simulink model "DAB_Tri_Trap"  (R2022b)
settings: Solver=ode23t  StartTime=0.0  StopTime=1/fsw*10000  MaxStep=1/100000  RelTol=1e-7  AbsTol=1e-7
StartFcn:
  | tic
StopFcn:
  | toc
undefined symbols (not defined in the file): DiscIntNeverNeededParam, fsw, L, n, ntemp, period, R_Load, tau, ts_pwm, Vdc1, Vth
libraries: nesl_utility x15, fl_lib x12, ee_lib x8, simulink x5, slpidlib x1
(part 1 of 2)
settings Model: Creator=jvansick  LastModifiedBy=jvansick
settings SolverCC: AutoScaleAbsTol=off  ExtrapolationOrder=1  ODENIntegrationMethod=ode14x
settings DebuggingCC: UnconnectedInputMsg=warning  UnconnectedOutputMsg=warning  UnconnectedLineMsg=warning
settings ModelReferenceCC: EnableRefExpFcnMdlSchedulingChecks=on
settings RTWCC: DLArmComputeVersion=19.05

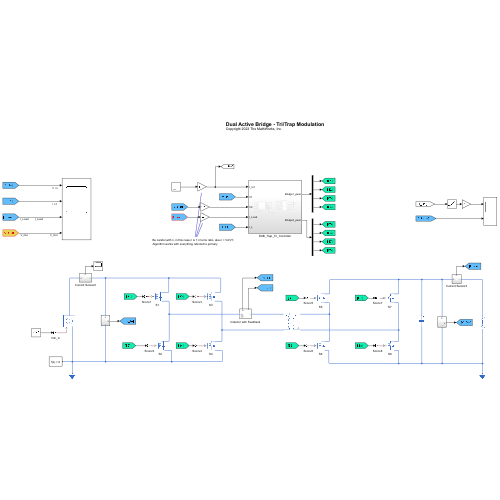
[thumbnail: Simulink's stored preview of the top-level diagram]
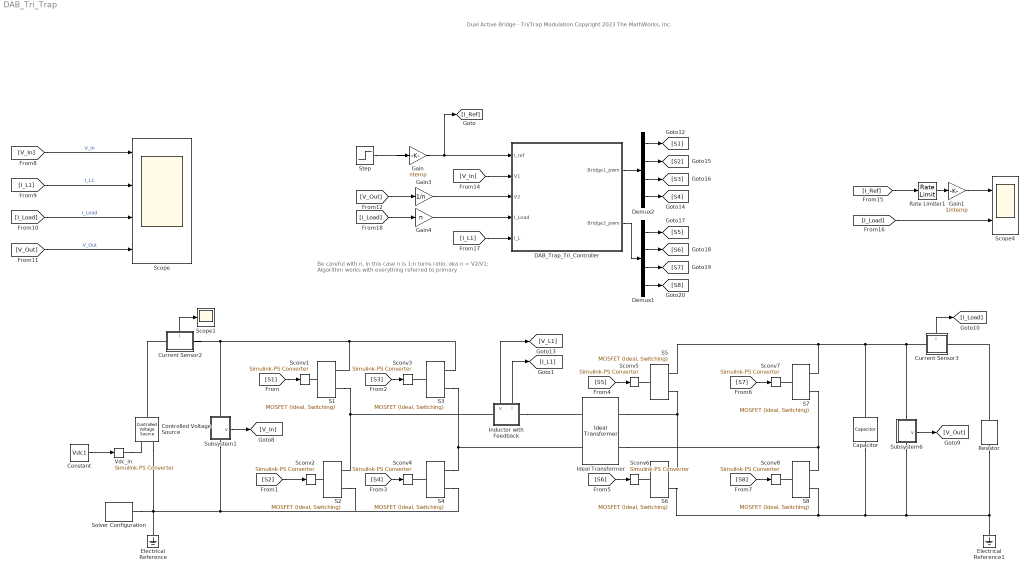
== system DAB_Tri_Trap ==
  note: Be careful with n, in this case n is 1:n turns ratio, aka n = V2/V1; Algorithm works with everything referred to primary
  note: Dual Active Bridge - Tri/Trap Modulation
      | Copyright 2023 The MathWorks, Inc.
  Capacitor : fl_lib/Electrical/Electrical Elements/Capacitor  c=Cout F  r=0 Ohm  g=0 1/Ohm  i_specify=off  i_priority=None  i=0 A  i_nominal_specify=off  i_nominal_unit=A  i_nominal_value=1  v_specify=off  v_priority=None  v=Vdc2 V  v_nominal_specify=off  v_nominal_unit=V  v_nominal_value=1  vc_specify=on  vc_priority=High  vc=Vdc2 V  vc_nominal_specify=off  vc_nominal_unit=V  vc_nominal_value=1
  Constant : Constant  Value=Vdc1
  Controlled Voltage Source : fl_lib/Electrical/Electrical Sources/Controlled Voltage Source
  Current Sensor2 : Subsystem
      settings: PortSchema="{\"entries\":[{\"content\":{\"sides\":[{\"content\":{\"connectorIds\":[\"LConn1\"]},\"type\":\"ConnectorPlacement.EquallySpacedRectSide\",\"uuid\":\"e9388151-e471-4783-81c5-5134e1313d7c\"},{\"content\":{\"connectorIds\":[\"RConn1\"],\"side\":\"RIGHT\"},\"type\":\"ConnectorPlacement.EquallySpacedRectSide\",\"uuid\":\"bcb23f28-0826-4736-ab91-150a314eb643\"},{\"content\":{\"connectorIds\":[\"Out1\"],\"side\":\"TOP\"},\"type\":\"ConnectorPlacement.EquallySpacedRectSide\",\"uuid\":\"e1937689-3337-4922-a316-f56c73fb0974\"}]},\"type\":\"ConnectorPlacement.EquallySpacedConnector\",\"uuid\":\"dc34a384-5aa5-46fc-88a5-47651899efae\"}],\"packageUris\":[\"http://schema.mathworks.com/mf0/Connector/R2020b\"],\"version\":\"1.0\"}"
  Current Sensor3 : Subsystem
      settings: PortSchema="{\"entries\":[{\"content\":{\"sides\":[{\"content\":{\"connectorIds\":[\"LConn1\"]},\"type\":\"ConnectorPlacement.EquallySpacedRectSide\",\"uuid\":\"e9388151-e471-4783-81c5-5134e1313d7c\"},{\"content\":{\"connectorIds\":[\"RConn1\"],\"side\":\"RIGHT\"},\"type\":\"ConnectorPlacement.EquallySpacedRectSide\",\"uuid\":\"bcb23f28-0826-4736-ab91-150a314eb643\"},{\"content\":{\"connectorIds\":[\"Out1\"],\"side\":\"TOP\"},\"type\":\"ConnectorPlacement.EquallySpacedRectSide\",\"uuid\":\"e1937689-3337-4922-a316-f56c73fb0974\"}]},\"type\":\"ConnectorPlacement.EquallySpacedConnector\",\"uuid\":\"dc34a384-5aa5-46fc-88a5-47651899efae\"}],\"packageUris\":[\"http://schema.mathworks.com/mf0/Connector/R2020b\"],\"version\":\"1.0\"}"
  DAB_Trap_Tri_Controller : Subsystem
  Demux1 : Demux
  Demux2 : Demux
  Electrical Reference : fl_lib/Electrical/Electrical Elements/Electrical Reference
  Electrical Reference1 : fl_lib/Electrical/Electrical Elements/Electrical Reference
  Gain : Gain  Gain=ntemp
  Gain1 : Gain  Gain=1/ntemp
  Gain3 : Gain  Gain=1/n
  Gain4 : Gain  Gain=n
  Ideal Transformer : fl_lib/Electrical/Electrical Elements/Ideal Transformer  n=1/n  i1_specify=off  i1_priority=None  i1=0 A  i1_nominal_specify=off  i1_nominal_unit=A  i1_nominal_value=1  v1_specify=off  v1_priority=None  v1=0 V  v1_nominal_specify=off  v1_nominal_unit=V  v1_nominal_value=1  i2_specify=off  i2_priority=None  i2=0 A  i2_nominal_specify=off  i2_nominal_unit=A  i2_nominal_value=1  v2_specify=off  v2_priority=None  v2=0 V  v2_nominal_specify=off  v2_nominal_unit=V  v2_nominal_value=1
  Inductor with Feedback : Subsystem  mask{L=L}
      mask prompts: L "Inductance"
      settings: PortSchema="{\"entries\":[{\"content\":{\"sides\":[{\"content\":{\"connectorIds\":[\"LConn1\"]},\"type\":\"ConnectorPlacement.EquallySpacedRectSide\",\"uuid\":\"d17b03de-5a5d-44ef-b1c9-12c97ac90336\"},{\"content\":{\"connectorIds\":[\"RConn1\"],\"side\":\"RIGHT\"},\"type\":\"ConnectorPlacement.EquallySpacedRectSide\",\"uuid\":\"dcf9dd19-1bc3-435d-be19-5082ce08996a\"},{\"content\":{\"connectorIds\":[\"Out1\",\"Out2\"],\"side\":\"TOP\"},\"type\":\"ConnectorPlacement.EquallySpacedRectSide\",\"uuid\":\"d1169a59-8047-479a-baab-e2604a43bf69\"}]},\"type\":\"ConnectorPlacement.EquallySpacedConnector\",\"uuid\":\"f70215f2-dcac-493e-85d0-6d9635986165\"}],\"packageUris\":[\"http://schema.mathworks.com/mf0/Connector/R2020b\"],\"version\":\"1.0\"}"
  Rate Limiter1 : RateLimiter  RisingSlewLimit=fsw/500  FallingSlewLimit=-fsw/500  SampleTimeMode=inherited  InitialCondition=15*ntemp
  Resistor : fl_lib/Electrical/Electrical Elements/Resistor  R=R_Load Ohm  i_specify=off  i_priority=None  i=0 A  i_nominal_specify=off  i_nominal_unit=A  i_nominal_value=1  v_specify=off  v_priority=None  v=0 V  v_nominal_specify=off  v_nominal_unit=V  v_nominal_value=1
  S{1..8} (8 alike) : ee_lib/Semiconductors & Converters/MOSFET (Ideal, Switching)  port_option=ee.enum.controlport.ps  Rds=R_ds Ohm  Goff=1e-5 1/Ohm  Vth=Vth V  diode_param=2  diode_Vf=V_fw_d V  diode_Ron=R_don Ohm  diode_Goff=1e-5 1/Ohm  diode_C=50e-9 F  diode_iRM=-235 A  diode_iF=300 A  diode_idot=-50 A/us  diode_trr_param=1  diode_trr_factor=3  diode_trr=15 us  diode_Qrr=1500 s*uA  ids_specify=off  ids_priority=None  ids=0 A  ids_nominal_specify=off  ids_nominal_unit=A  ids_nominal_value=1  vds_specify=off  vds_priority=None  vds=0 V  vds_nominal_specify=off  vds_nominal_unit=V  vds_nominal_value=1  vgs_specify=off  vgs_priority=None  vgs=0 V  vgs_nominal_specify=off  vgs_nominal_unit=V  vgs_nominal_value=1  thermal_loss_option=ee.enum.converters.thermalLossOption.constantvalues  Von_data=[0, 1.8, 3.2, 6, 10, 16; 0, 2, 5.5, 9.5, 15, 25] V  Tj=[298.15, 448.15] K  Iout_data=[0, 20, 40, 60, 80, 100] A  Eon_data=[0, 55.04, 124.57, 235.53, 362.12; 0, 71.25, 161.25, 304.88, 468.75] * 1e-6 J  Eoff_data=[0, 18, 30, 56.1, 76.5; 0, 22.5, 37.5, 70.13, 95.63] * 1e-6 J  Tj_loss=[298.15, 448.15] K  Iout_data_loss=[0, 10, 20, 30, 40] A  Eon_scalar=22.86e-3 J  Eoff_scalar=17.14e-3 J  Voff=300 V  Iout_scalar=600 A  diodeModelType=ee.enum.converters.diodeModelType.pwl  diodeTableType=ee.enum.diode.tableType.IfMat  diode_IfMat=[.07, .12, .19, 1.75, 4.24, 7.32, 11.2; .16, .3, .72, 2.14, 4.02, 6.35, 9.12] A  diode_VfMat=[.9, 1.15, 1.25, 1.5, 1.75, 2.17, 2.6, 2.85; .58, .68, .75, 1.1, 1.38, 1.77, 2.27, 2.7] V  diode_TjVec=[25, 125] degC  diode_VfVec=[.5, .7, .9, 1.3, 1.7, 2.1, 2.5] V  diode_IfVec=[.1, .2, .5, 1, 2, 4, 7, 10] A  diode_Vr=-600 V  diode_Ls=150 nH  diode_Erec=0.03 J  thermal_network_parameterization=ee.enum.thermalNetworkTopology.external  Rth=[.03, .2] K/W  Rth_Cauer=[.03, .1, .2] K/W  Rth_Foster=[.03, .2] K/W  thermal_mass_parameterization=ee.enum.thermalNetwork.timeconstant  thermal_mass=[3, 25] J/K  thermal_mass_Cauer=[3, 10, 25] J/K  thermal_mass_Foster=[33, 50] J/K  thermal_time_constant=[.1, 5] s  thermal_time_constant_Cauer=[.1, 1, 5] s  thermal_time_constant_Foster=[1, 10] s  thermal_mass_initial_temperatures=[25, 25] degC  thermal_mass_initial_temperatures_Cauer=[25, 25, 25] degC  junction_thermal_mass=0.1 J/K  Tvec_initial_Foster=[25, 25, 25, 25] degC  no_thermal_network=0  junction_temperature_specify=off  junction_temperature_priority=None  junction_temperature=25 degC  junction_temperature_nominal_specify=off  junction_temperature_nominal_unit=degC  junction_temperature_nominal_value=1  Qj_specify=off  Qj_priority=None  Qj=0 W  Qj_nominal_specify=off  Qj_nominal_unit=W  Qj_nominal_value=1
  Sconv{1..8} (8 alike) : nesl_utility/Simulink-PS Converter  PhysicalDomain=network_engine_domain  SubClassName=ps_input  LeftPortType=input  RightPortType=output  PseudoPeriodic=off  Frequencies=[]  NoiseDistribution=none  NoiseParameters=[]  Unit=1  AffineConversion=off  FilteringAndDerivatives=provide  SimscapeFilterOrder=1  InputFilterTimeConstant=0.001  UdotUserProvided=0
  Scope : Scope  NumInputPorts=4
  Scope1 : Scope
  Scope4 : Scope  NumInputPorts=2
  Solver Configuration : nesl_utility/Solver Configuration  PhysicalDomain=network_engine_domain  SubClassName=solver  LeftPortType=input  RightPortType=generic  Tones=[]  Harmonics=[]  SimulateNoise=off  Profile=off  UseLocalSampling=off  EnableSwitchedLinearOptims=on  FrequencyDomain=off  UseCCode=off  RelTol=0.001  AbsTol=1e-06  MinStep=1e-09  ToWorkspace=off  RevertToSquareIcSolve=off  NumHomotopyIterations=100  PhasorMode=off  PhasorModeNumHarmonics=1  ConsistencySolver=NEWTON_FTOL  IndexReductionMethod=DerivativeReplacement  DoDC=off  ResidualTolerance=1e-09  ConsistencyTolSource=GLOBAL  ConsistencyAbsTol=0.001  ConsistencyRelTol=0.001  ConsistencyTolFactor=0.001  UseLocalSolver=off  LocalSolverChoice=NE_BACKWARD_EULER_ADVANCER  ResolveIndetEquations=on  FunctionEvalNumThread=1  LocalSolverSampleTime=0.001  DoFixedCost=off  MaxNonlinIter=3  MaxModeIter=2  ComputeImpulses=off  ImpulseIterations=2  LinearAlgebra=auto  LinearAlgebraNumThread=0  EquationFormulation=NE_TIME_EF  DelaysMemoryBudget=1024  AutomaticFiltering=on  FilteringTimeConstant=0.001  PartitionStorageMethod=AS_NEEDED  PartitionMemoryBudget=1024  PartitionMethod=ROBUST
  Step : Step  Time=1/fsw*5000  Before=15.25  After=19.35  SampleTime=1/fsw
  Subsystem1 : Subsystem
      settings: PortSchema="{\"entries\":[{\"content\":{\"sides\":[{\"content\":{\"connectorIds\":[\"LConn1\"]},\"type\":\"ConnectorPlacement.EquallySpacedRectSide\",\"uuid\":\"e9388151-e471-4783-81c5-5134e1313d7c\"},{\"content\":{\"connectorIds\":[\"RConn1\"],\"side\":\"RIGHT\"},\"type\":\"ConnectorPlacement.EquallySpacedRectSide\",\"uuid\":\"bcb23f28-0826-4736-ab91-150a314eb643\"},{\"content\":{\"connectorIds\":[\"Out1\"],\"side\":\"TOP\"},\"type\":\"ConnectorPlacement.EquallySpacedRectSide\",\"uuid\":\"e1937689-3337-4922-a316-f56c73fb0974\"}]},\"type\":\"ConnectorPlacement.EquallySpacedConnector\",\"uuid\":\"dc34a384-5aa5-46fc-88a5-47651899efae\"}],\"packageUris\":[\"http://schema.mathworks.com/mf0/Connector/R2020b\"],\"version\":\"1.0\"}"
  Subsystem6 : Subsystem
      settings: PortSchema="{\"entries\":[{\"content\":{\"sides\":[{\"content\":{\"connectorIds\":[\"LConn1\"]},\"type\":\"ConnectorPlacement.EquallySpacedRectSide\",\"uuid\":\"e9388151-e471-4783-81c5-5134e1313d7c\"},{\"content\":{\"connectorIds\":[\"RConn1\"],\"side\":\"RIGHT\"},\"type\":\"ConnectorPlacement.EquallySpacedRectSide\",\"uuid\":\"bcb23f28-0826-4736-ab91-150a314eb643\"},{\"content\":{\"connectorIds\":[\"Out1\"],\"side\":\"TOP\"},\"type\":\"ConnectorPlacement.EquallySpacedRectSide\",\"uuid\":\"e1937689-3337-4922-a316-f56c73fb0974\"}]},\"type\":\"ConnectorPlacement.EquallySpacedConnector\",\"uuid\":\"dc34a384-5aa5-46fc-88a5-47651899efae\"}],\"packageUris\":[\"http://schema.mathworks.com/mf0/Connector/R2020b\"],\"version\":\"1.0\"}"
  Vdc_in : nesl_utility/Simulink-PS Converter  PhysicalDomain=network_engine_domain  SubClassName=ps_input  LeftPortType=input  RightPortType=output  PseudoPeriodic=off  Frequencies=[]  NoiseDistribution=none  NoiseParameters=[]  Unit=1  AffineConversion=off  FilteringAndDerivatives=provide  SimscapeFilterOrder=1  InputFilterTimeConstant=0.001  UdotUserProvided=0
  wires:
  [S1] -> Sconv1/1
  [S2] -> Sconv2/1
  [S3] -> Sconv3/1
  [S4] -> Sconv4/1
  [S6] -> Sconv6/1
  [S7] -> Sconv7/1
  [S8] -> Sconv8/1
  [S5] -> Sconv5/1
  Constant/1 -> Vdc_in/1
  Subsystem1/1(v) -> [V_In]
  [V_In] -> Scope/1  "V_in"
  [I_L1] -> Scope/2  "I_L1"
  [I_Load] -> Scope/3  "I_Load"
  Current Sensor2/1(i) -> Scope1/1
  [V_Out] -> Scope/4  "V_Out"
  Demux2/1 -> [S1]
  Demux2/4 -> [S4]
  Demux2/2 -> [S2]
  Demux2/3 -> [S3]
  Demux1/1 -> [S5]
  Demux1/2 -> [S6]
  Demux1/3 -> [S7]
  Demux1/4 -> [S8]
  DAB_Trap_Tri_Controller/2(Bridge2_pwm) -> Demux1/1
  DAB_Trap_Tri_Controller/1(Bridge1_pwm) -> Demux2/1
  Current Sensor3/1(i) -> [I_Load]
  Subsystem6/1(v) -> [V_Out]
  Step/1 -> Gain/1
  [V_Out] -> Gain3/1
  [V_In] -> DAB_Trap_Tri_Controller/2(V1)
  [I_L1] -> DAB_Trap_Tri_Controller/5(I_L)
  [I_Load] -> Gain4/1
  [I_Load] -> Scope4/2
  [I_Ref] -> Rate Limiter1/1
  Rate Limiter1/1 -> Gain1/1
  Gain/1 -> [I_Ref], DAB_Trap_Tri_Controller/1(I_ref)
  Gain3/1 -> DAB_Trap_Tri_Controller/3(V2)
  Gain4/1 -> DAB_Trap_Tri_Controller/4(I_Load)
  Inductor with Feedback/1(v) -> [V_L1]
  Inductor with Feedback/2(i) -> [I_L1]
  Gain1/1 -> Scope4/1
  connections:
  Subsystem1/LConn1 -- Current Sensor2/RConn1 -- S1/RConn1 -- S3/RConn1
  Controlled Voltage Source/RConn2 -- Electrical Reference/LConn1 -- S4/RConn2 -- S2/RConn2 -- Subsystem1/RConn1 -- Solver Configuration/RConn1
  Vdc_in/RConn1 -- Controlled Voltage Source/RConn1
  S2/LConn1 -- Sconv2/RConn1
  Sconv1/RConn1 -- S1/LConn1
  S3/LConn1 -- Sconv3/RConn1
  S4/LConn1 -- Sconv4/RConn1
  S6/LConn1 -- Sconv6/RConn1
  S8/LConn1 -- Sconv8/RConn1
  S7/LConn1 -- Sconv7/RConn1
  S5/LConn1 -- Sconv5/RConn1
  S3/RConn2 -- S4/RConn1 -- Ideal Transformer/LConn2
  S5/RConn2 -- Ideal Transformer/RConn1 -- S6/RConn1
  S7/RConn2 -- Ideal Transformer/RConn2 -- S8/RConn1
  Electrical Reference1/LConn1 -- S8/RConn2 -- S6/RConn2 -- Capacitor/RConn1 -- Subsystem6/RConn1 -- Resistor/RConn1
  Current Sensor2/LConn1 -- Controlled Voltage Source/LConn1
  S5/RConn1 -- S7/RConn1 -- Capacitor/LConn1 -- Subsystem6/LConn1 -- Current Sensor3/LConn1
  Resistor/LConn1 -- Current Sensor3/RConn1
  S2/RConn1 -- Inductor with Feedback/LConn1 -- S1/RConn2
  Inductor with Feedback/RConn1 -- Ideal Transformer/LConn1

== system DAB_Tri_Trap/Current Sensor2 ==
  Current Sensor : fl_lib/Electrical/Electrical Sensors/Current Sensor
  PS-Simulink Converter1 : nesl_utility/PS-Simulink Converter  PhysicalDomain=network_engine_domain  SubClassName=ps_output  LeftPortType=input  RightPortType=output  PseudoPeriodic=off  Frequencies=[]  VectorFormat=1-D array  Unit=inherit  AffineConversion=off
  + : PMIOPort  Side=Left
  - : PMIOPort  Port=2  Side=Right
  i : Outport
  wires:
  PS-Simulink Converter1/1 -> i/1
  connections:
  Current Sensor/RConn2 -- -/RConn1
  Current Sensor/LConn1 -- +/RConn1
  Current Sensor/RConn1 -- PS-Simulink Converter1/LConn1

== system DAB_Tri_Trap/Current Sensor3 ==
  Current Sensor : fl_lib/Electrical/Electrical Sensors/Current Sensor
  PS-Simulink Converter1 : nesl_utility/PS-Simulink Converter  PhysicalDomain=network_engine_domain  SubClassName=ps_output  LeftPortType=input  RightPortType=output  PseudoPeriodic=off  Frequencies=[]  VectorFormat=1-D array  Unit=inherit  AffineConversion=off
  + : PMIOPort  Side=Left
  - : PMIOPort  Port=2  Side=Right
  i : Outport
  wires:
  PS-Simulink Converter1/1 -> i/1
  connections:
  Current Sensor/RConn1 -- PS-Simulink Converter1/LConn1
  Current Sensor/LConn1 -- +/RConn1
  Current Sensor/RConn2 -- -/RConn1

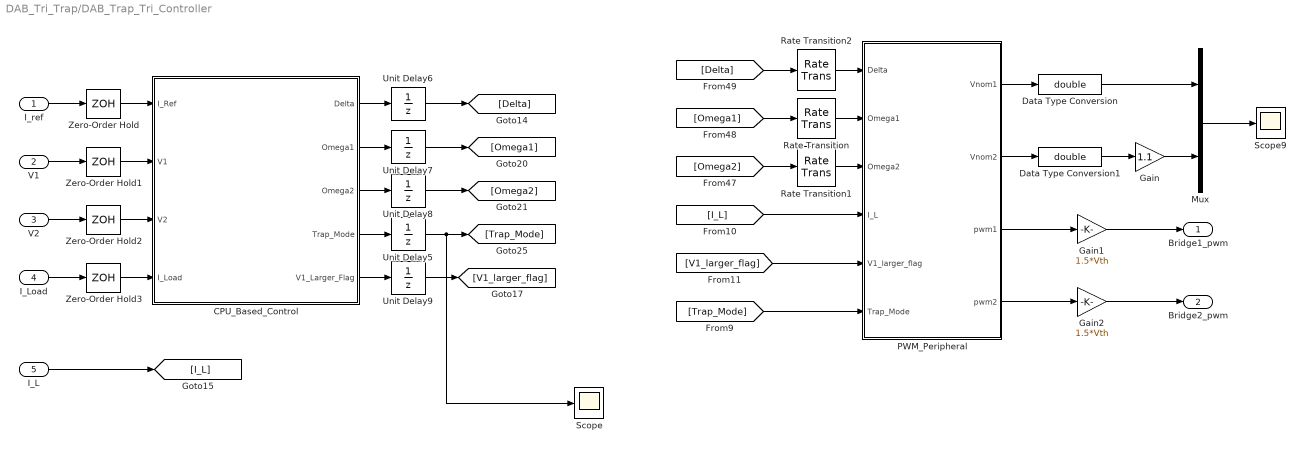
== system DAB_Tri_Trap/DAB_Trap_Tri_Controller ==
  I_ref : Inport
  V1 : Inport  Port=2
  V2 : Inport  Port=3
  I_Load : Inport  Port=4
  I_L : Inport  Port=5
  CPU_Based_Control : Subsystem
  Data Type Conversion : DataTypeConversion  OutDataTypeStr=double  SaturateOnIntegerOverflow=off  RndMeth=Floor
  Data Type Conversion1 : DataTypeConversion  OutDataTypeStr=double  SaturateOnIntegerOverflow=off  RndMeth=Floor
  Gain : Gain  Gain=1.1
  Gain1 : Gain  Gain=1.5*Vth
  Gain2 : Gain  Gain=1.5*Vth
  Mux : Mux  Inputs=2
  PWM_Peripheral : Subsystem
  Rate Transition : RateTransition  OutPortSampleTime=period
  Rate Transition1 : RateTransition  OutPortSampleTime=period
  Rate Transition2 : RateTransition  OutPortSampleTime=period
  Scope : Scope
  Scope9 : Scope
  Unit Delay{5..9} (5 alike) : UnitDelay  SampleTime=period  HasFrameUpgradeWarning=on
  Zero-Order Hold{,1..3} (4 alike) : ZeroOrderHold  SampleTime=period
  Bridge1_pwm : Outport
  Bridge2_pwm : Outport  Port=2
  wires:
  Data Type Conversion1/1 -> Gain/1
  Data Type Conversion/1 -> Mux/1
  Rate Transition2/1 -> PWM_Peripheral/1(Delta)
  Rate Transition1/1 -> PWM_Peripheral/3(Omega2)
  Rate Transition/1 -> PWM_Peripheral/2(Omega1)
  PWM_Peripheral/4(pwm2) -> Gain2/1
  PWM_Peripheral/3(pwm1) -> Gain1/1
  [Delta] -> Rate Transition2/1
  Mux/1 -> Scope9/1
  PWM_Peripheral/1(Vnom1) -> Data Type Conversion/1
  Gain/1 -> Mux/2
  PWM_Peripheral/2(Vnom2) -> Data Type Conversion1/1
  [Omega1] -> Rate Transition/1
  [Omega2] -> Rate Transition1/1
  V2/1 -> Zero-Order Hold2/1
  V1/1 -> Zero-Order Hold1/1
  [I_L] -> PWM_Peripheral/4(I_L)
  [V1_larger_flag] -> PWM_Peripheral/5(V1_larger_flag)
  [Trap_Mode] -> PWM_Peripheral/6(Trap_Mode)
  I_Load/1 -> Zero-Order Hold3/1
  I_L/1 -> [I_L]
  I_ref/1 -> Zero-Order Hold/1
  Zero-Order Hold1/1 -> CPU_Based_Control/2(V1)
  Zero-Order Hold2/1 -> CPU_Based_Control/3(V2)
  Zero-Order Hold3/1 -> CPU_Based_Control/4(I_Load)
  CPU_Based_Control/4(Trap_Mode) -> Unit Delay5/1
  CPU_Based_Control/1(Delta) -> Unit Delay6/1
  CPU_Based_Control/2(Omega1) -> Unit Delay7/1
  CPU_Based_Control/3(Omega2) -> Unit Delay8/1
  CPU_Based_Control/5(V1_Larger_Flag) -> Unit Delay9/1
  Zero-Order Hold/1 -> CPU_Based_Control/1(I_Ref)
  Unit Delay5/1 -> Scope/1, [Trap_Mode]
  Unit Delay6/1 -> [Delta]
  Unit Delay7/1 -> [Omega1]
  Unit Delay8/1 -> [Omega2]
  Unit Delay9/1 -> [V1_larger_flag]
  Gain1/1 -> Bridge1_pwm/1
  Gain2/1 -> Bridge2_pwm/1

== system DAB_Tri_Trap/Inductor with Feedback ==
  note: Subsystem2
  Gain : Gain  Gain=1/L
  Integrator : Integrator
  L1 : fl_lib/Electrical/Electrical Elements/Inductor  l=L H  r=.1 Ohm  g=0 1/Ohm  i_specify=off  i_priority=None  i=0 A  i_nominal_specify=off  i_nominal_unit=A  i_nominal_value=1  v_specify=off  v_priority=None  v=0 V  v_nominal_specify=off  v_nominal_unit=V  v_nominal_value=1  i_L_specify=off  i_L_priority=High  i_L=0 A  i_L_nominal_specify=off  i_L_nominal_unit=A  i_L_nominal_value=1
  PS-Simulink Converter : nesl_utility/PS-Simulink Converter  PhysicalDomain=network_engine_domain  SubClassName=ps_output  LeftPortType=input  RightPortType=output  PseudoPeriodic=off  Frequencies=[]  VectorFormat=1-D array  Unit=inherit  AffineConversion=off
  Voltage Sensor : fl_lib/Electrical/Electrical Sensors/Voltage Sensor
  + : PMIOPort  Side=Left
  - : PMIOPort  Port=2  Side=Right
  v : Outport
  i : Outport  Port=2
  wires:
  PS-Simulink Converter/1 -> v/1, Integrator/1
  Gain/1 -> i/1
  Integrator/1 -> Gain/1
  connections:
  L1/RConn1 -- -/RConn1 -- Voltage Sensor/RConn2
  +/RConn1 -- L1/LConn1 -- Voltage Sensor/LConn1
  Voltage Sensor/RConn1 -- PS-Simulink Converter/LConn1

== system DAB_Tri_Trap/Subsystem1 ==
  PS-Simulink Converter : nesl_utility/PS-Simulink Converter  PhysicalDomain=network_engine_domain  SubClassName=ps_output  LeftPortType=input  RightPortType=output  PseudoPeriodic=off  Frequencies=[]  VectorFormat=1-D array  Unit=inherit  AffineConversion=off
  Voltage Sensor : fl_lib/Electrical/Electrical Sensors/Voltage Sensor
  + : PMIOPort  Side=Left
  - : PMIOPort  Port=2  Side=Right
  v : Outport
  wires:
  PS-Simulink Converter/1 -> v/1
  connections:
  Voltage Sensor/RConn2 -- -/RConn1
  Voltage Sensor/RConn1 -- PS-Simulink Converter/LConn1
  Voltage Sensor/LConn1 -- +/RConn1

== system DAB_Tri_Trap/Subsystem6 ==
  PS-Simulink Converter : nesl_utility/PS-Simulink Converter  PhysicalDomain=network_engine_domain  SubClassName=ps_output  LeftPortType=input  RightPortType=output  PseudoPeriodic=off  Frequencies=[]  VectorFormat=1-D array  Unit=inherit  AffineConversion=off
  Voltage Sensor : fl_lib/Electrical/Electrical Sensors/Voltage Sensor
  + : PMIOPort  Side=Left
  - : PMIOPort  Port=2  Side=Right
  v : Outport
  wires:
  PS-Simulink Converter/1 -> v/1
  connections:
  Voltage Sensor/LConn1 -- +/RConn1
  Voltage Sensor/RConn1 -- PS-Simulink Converter/LConn1
  Voltage Sensor/RConn2 -- -/RConn1

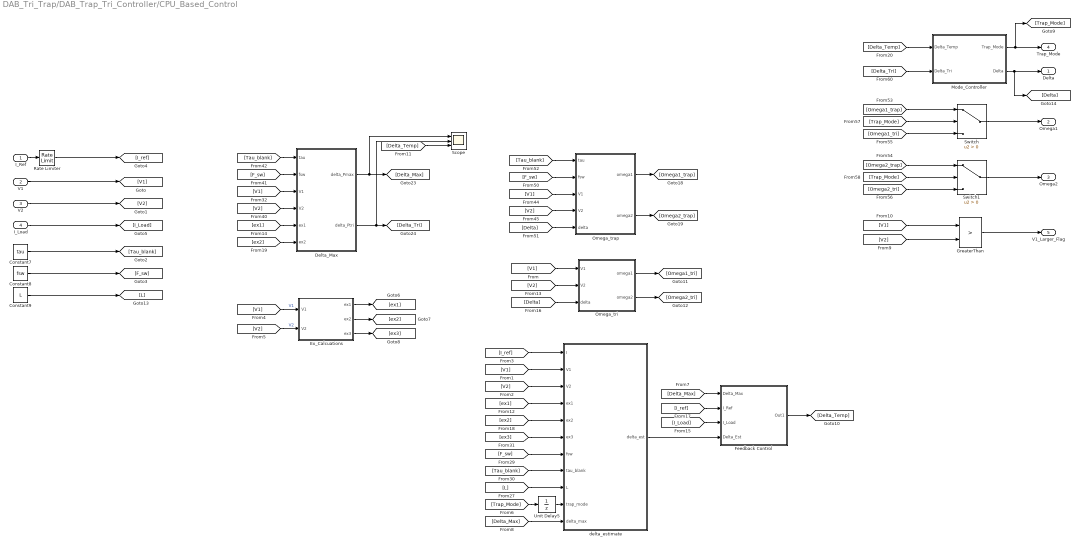
== system DAB_Tri_Trap/DAB_Trap_Tri_Controller/CPU_Based_Control ==
  I_Ref : Inport
  V1 : Inport  Port=2
  V2 : Inport  Port=3
  I_Load : Inport  Port=4
  Constant7 : Constant  Value=tau
  Constant8 : Constant  Value=fsw
  Constant9 : Constant  Value=L
  Delta_Max : MATLAB Function  TreatAsAtomicUnit=on
  Ex_Calcuations : Subsystem
  Feedback Control : Subsystem
  GreaterThan : RelationalOperator  Operator=>  OutDataTypeStr=boolean  RndMeth=Simplest  InputSameDT=off
  Mode_Controller : Subsystem
  Omega_trap : MATLAB Function  TreatAsAtomicUnit=on
  Omega_tri : MATLAB Function  TreatAsAtomicUnit=on
  Rate Limiter : RateLimiter  RisingSlewLimit=fsw/500  FallingSlewLimit=-fsw/500  SampleTimeMode=inherited  InitialCondition=15*ntemp
  Scope : Scope  NumInputPorts=3
  Switch : Switch  Criteria=u2 > Threshold  SaturateOnIntegerOverflow=off  InputSameDT=off
  Switch1 : Switch  Criteria=u2 > Threshold  SaturateOnIntegerOverflow=off  InputSameDT=off
  Unit Delay5 : UnitDelay  SampleTime=period  HasFrameUpgradeWarning=on
  delta_estimate : MATLAB Function  TreatAsAtomicUnit=on
  Delta : Outport
  Omega1 : Outport  Port=2
  Omega2 : Outport  Port=3
  Trap_Mode : Outport  Port=4
  V1_Larger_Flag : Outport  Port=5
  wires:
  [V1] -> Omega_trap/3(V1)
  Delta_Max/1(delta_Pmax) -> Scope/1, [Delta_Max]
  [Omega1_tri] -> Switch/3
  [V1] -> Omega_tri/1(V1)
  [ex2] -> delta_estimate/5(ex2)
  [ex1] -> delta_estimate/4(ex1)
  [Tau_blank] -> delta_estimate/8(tau_blank)
  [L] -> delta_estimate/9(L)
  [F_sw] -> delta_estimate/7(fsw)
  Delta_Max/2(delta_Ptri) -> Scope/2, [Delta_Tri]
  [V1] -> delta_estimate/2(V1)
  [V2] -> Omega_tri/2(V2)
  Omega_tri/2(omega2) -> [Omega2_tri]
  [V2] -> delta_estimate/3(V2)
  [ex2] -> Delta_Max/6(ex2)
  Omega_tri/1(omega1) -> [Omega1_tri]
  GreaterThan/1 -> V1_Larger_Flag/1
  Omega_trap/1(omega1) -> [Omega1_trap]
  [Delta] -> Omega_tri/3(delta)
  [V1] -> Delta_Max/3(V1)
  [I_ref] -> delta_estimate/1(I)
  [V2] -> Delta_Max/4(V2)
  [ex1] -> Delta_Max/5(ex1)
  [Delta_Max] -> delta_estimate/11(delta_max)
  [V2] -> Omega_trap/4(V2)
  [F_sw] -> Omega_trap/2(fsw)
  [ex3] -> delta_estimate/6(ex3)
  [Omega2_trap] -> Switch1/1
  [Tau_blank] -> Delta_Max/1(tau)
  [Delta] -> Omega_trap/5(delta)
  [Tau_blank] -> Omega_trap/1(tau)
  [F_sw] -> Delta_Max/2(fsw)
  [Omega1_trap] -> Switch/1
  [Trap_Mode] -> Switch/2
  [Trap_Mode] -> Unit Delay5/1
  [Omega2_tri] -> Switch1/3
  Ex_Calcuations/2(ex2) -> [ex2]
  Omega_trap/2(omega2) -> [Omega2_trap]
  [Trap_Mode] -> Switch1/2
  Constant8/1 -> [F_sw]
  Ex_Calcuations/1(ex1) -> [ex1]
  Ex_Calcuations/3(ex3) -> [ex3]
  [V2] -> Ex_Calcuations/2(V2)  "V2"
  [V1] -> Ex_Calcuations/1(V1)  "V1"
  Constant7/1 -> [Tau_blank]
  Unit Delay5/1 -> delta_estimate/10(trap_mode)
  I_Ref/1 -> Rate Limiter/1
  Switch/1 -> Omega1/1
  Switch1/1 -> Omega2/1
  [Delta_Temp] -> Mode_Controller/1(Delta_Temp)
  [Delta_Tri] -> Mode_Controller/2(Delta_Tri)
  Mode_Controller/1(Trap_Mode) -> [Trap_Mode], Trap_Mode/1
  Mode_Controller/2(Delta) -> [Delta], Delta/1
  [Delta_Max] -> Feedback Control/1(Delta_Max)
  [I_ref] -> Feedback Control/2(I_Ref)
  [I_Load] -> Feedback Control/3(I_Load)
  delta_estimate/1(delta_est) -> Feedback Control/4(Delta_Est)
  [V2] -> GreaterThan/2
  [V1] -> GreaterThan/1
  [Delta_Temp] -> Scope/3
  Constant9/1 -> [L]
  V1/1 -> [V1]
  I_Load/1 -> [I_Load]
  Rate Limiter/1 -> [I_ref]
  V2/1 -> [V2]
  Feedback Control/1(Out1) -> [Delta_Temp]

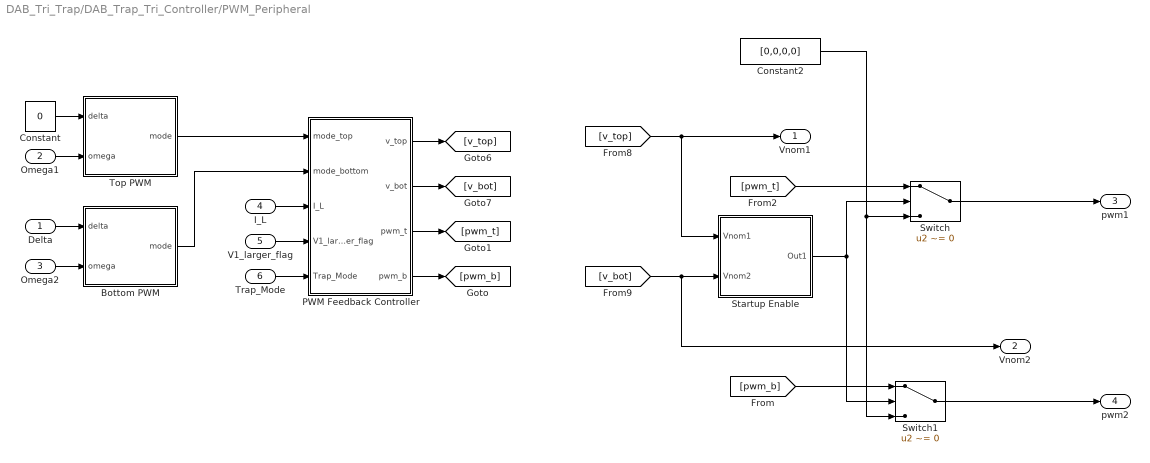
== system DAB_Tri_Trap/DAB_Trap_Tri_Controller/PWM_Peripheral ==
  Delta : Inport
  Omega1 : Inport  Port=2
  Omega2 : Inport  Port=3
  I_L : Inport  Port=4
  V1_larger_flag : Inport  Port=5
  Trap_Mode : Inport  Port=6
  Bottom PWM : Subsystem
  Constant : Constant  Value=0  SampleTime=ts_pwm
  Constant2 : Constant  Value=[0,0,0,0]  SampleTime=ts_pwm
  PWM Feedback Controller : Subsystem
  Startup Enable : Subsystem
  Switch : Switch  Criteria=u2 ~= 0  SaturateOnIntegerOverflow=off  InputSameDT=off
  Switch1 : Switch  Criteria=u2 ~= 0  SaturateOnIntegerOverflow=off  InputSameDT=off
  Top PWM : Subsystem
  Vnom1 : Outport
  Vnom2 : Outport  Port=2
  pwm1 : Outport  Port=3
  pwm2 : Outport  Port=4
  wires:
  Startup Enable/1(Out1) -> Switch1/2, Switch/2
  Switch1/1 -> pwm2/1
  Constant2/1 -> Switch1/3, Switch/3
  Switch/1 -> pwm1/1
  [v_bot] -> Vnom2/1, Startup Enable/2(Vnom2)
  Constant/1 -> Top PWM/1(delta)
  Omega2/1 -> Bottom PWM/2(omega)
  Delta/1 -> Bottom PWM/1(delta)
  [v_top] -> Vnom1/1, Startup Enable/1(Vnom1)
  Omega1/1 -> Top PWM/2(omega)
  [pwm_t] -> Switch/1
  [pwm_b] -> Switch1/1
  Top PWM/1(mode) -> PWM Feedback Controller/1(mode_top)
  Bottom PWM/1(mode) -> PWM Feedback Controller/2(mode_bottom)
  PWM Feedback Controller/1(v_top) -> [v_top]
  PWM Feedback Controller/2(v_bot) -> [v_bot]
  PWM Feedback Controller/3(pwm_t) -> [pwm_t]
  PWM Feedback Controller/4(pwm_b) -> [pwm_b]
  I_L/1 -> PWM Feedback Controller/3(I_L)
  V1_larger_flag/1 -> PWM Feedback Controller/4(V1_larger_flag)
  Trap_Mode/1 -> PWM Feedback Controller/5(Trap_Mode)

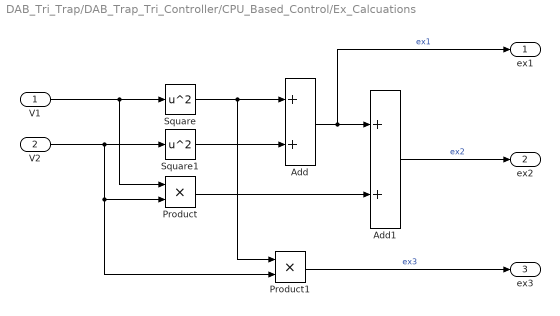
== system DAB_Tri_Trap/DAB_Trap_Tri_Controller/CPU_Based_Control/Ex_Calcuations ==
  V1 : Inport
  V2 : Inport  Port=2
  Add : Sum
  Add1 : Sum
  Product : Product
  Product1 : Product
  Square : Math  Operator=square
  Square1 : Math  Operator=square
  ex1 : Outport
  ex2 : Outport  Port=2
  ex3 : Outport  Port=3
  wires:
  Square1/1 -> Add/2
  Add/1 -> ex1/1, Add1/1  "ex1"
  Product1/1 -> ex3/1  "ex3"
  V2/1 -> Square1/1, Product/2, Product1/2
  Product/1 -> Add1/2
  V1/1 -> Square/1, Product/1
  Square/1 -> Add/1, Product1/1
  Add1/1 -> ex2/1  "ex2"

== system DAB_Tri_Trap/DAB_Trap_Tri_Controller/CPU_Based_Control/Feedback Control ==
  Delta_Max : Inport
  I_Ref : Inport  Port=2
  I_Load : Inport  Port=3
  Delta_Est : Inport  Port=4
  Add2 : Sum
  Gain2 : Gain
  Min : MinMax  Inputs=2
  PID Controller : slpidlib/PID Controller  Controller=PID  Form=Parallel  TimeDomain=Discrete-time  UseExternalTs=off  SampleTime=-1  IntegratorMethod=Forward Euler  FilterMethod=Forward Euler  ControllerParametersSource=internal  P=1  I=6  UseKiTs=off  D=0.002  N=20  UseFilter=on  TunerSelectOption=Transfer Function Based (PID Tuner App)  InitialConditionSource=internal  InitialConditionForIntegrator=0  InitialConditionForFilter=0  DifferentiatorICPrevScaledInput=0  ExternalReset=none  TrackingMode=off  Kt=1  LimitOutput=on  SatLimitsSource=internal  UpperSaturationLimit=pi/4  LowerSaturationLimit=-pi/4  LinearizeAsGain=on  AntiWindupMode=clamping  Kb=1  LimitIntegrator=off  UpperIntegratorSaturationLimit=inf  LowerIntegratorSaturationLimit=-inf  POutMin=[]  POutMax=[]  IOutMin=[]  IOutMax=[]  DOutMin=[]  DOutMax=[]  NOutMin=[]  NOutMax=[]  SumOutMin=[]  SumOutMax=[]  SaturationOutMin=[]  SaturationOutMax=[]  PParamMin=[]  PParamMax=[]  IParamMin=[]  IParamMax=[]  DParamMin=[]  DParamMax=[]  NParamMin=[]  NParamMax=[]  KbParamMin=[]  KbParamMax=[]  KtParamMin=[]  KtParamMax=[]  KbOutMin=[]  KbOutMax=[]  KtOutMin=[]  KtOutMax=[]  IntegratorOutMin=[]  IntegratorOutMax=[]  FilterOutMin=[]  FilterOutMax=[]  SumI1OutMin=[]  SumI1OutMax=[]  SumI2OutMin=[]  SumI2OutMax=[]  SumI3OutMin=[]  SumI3OutMax=[]  SumI4OutMin=[]  SumI4OutMax=[]  SumDOutMin=[]  SumDOutMax=[]  DifferentiatorOutMin=[]  DifferentiatorOutMax=[]  FilterDiffOutCoefMin=[]  FilterDiffOutCoefMax=[]  ReciprocalOutMin=[]  ReciprocalOutMax=[]  SumDenOutMin=[]  SumDenOutMax=[]  SumNumOutMin=[]  SumNumOutMax=[]  DivideOutMin=[]  DivideOutMax=[]  UdiffTsProdOutMin=[]  UdiffTsProdOutMax=[]  NTsProdOutMin=[]  NTsProdOutMax=[]  UintegralTsProdOutMin=[]  UintegralTsProdOutMax=[]  UngainTsProdOutMin=[]  UngainTsProdOutMax=[]  ClampingZeroOutDataTypeStr=Inherit: Inherit via back propagation  ClampingZeroOutMin=[]  ClampingZeroOutMax=[]  FilterDenConstantOutDataTypeStr=Inherit: Inherit via back propagation  FilterDenConstantOutMin=[]  FilterDenConstantOutMax=[]  PCopyOutDataTypeStr=Inherit: Inherit via back propagation  PCopyOutMin=[]  PCopyOutMax=[]  NCopyOutDataTypeStr=Inherit: Inherit via back propagation  NCopyOutMin=[]  NCopyOutMax=[]  IntegratorContinuousStateAttributes=''  IntegratorStateMustResolveToSignalObject=off  IntegratorRTWStateStorageClass=Auto  FilterContinuousStateAttributes=''  FilterStateMustResolveToSignalObject=off  FilterRTWStateStorageClass=Auto  ParallelPVariant=InternalParameters  IdealPVariant=Disabled  IVariant=InternalParameters  DVariant=InternalParameters  IntegratorVariant=Discrete  SatVariant=Enabled  AWVariant=DiscClampingParallel  PCopyVariant=Disabled  TRVariant=Disabled  FdbkBlocksVariant=Forward  IdealPFdbkVariant=Disabled  SatFdbkVariant=Disabled  DerivativeFilterVariant=ForwardEulerFilter  NVariant=InternalParameters  NCopyVariant=Disabled  FilterICVariant=InternalICsFilter  IntegratorICVariant=InternalICs  ExternalResetVariant=Disabled  TRSumVariant=Passthrough  SumFdbkVariant=Disabled  SumVariant=Sum_PID  TsampFilterVariant=InternalTs  TsampNgainVariant=Passthrough  TsampIntegralVariant=Passthrough  ExternalSaturationOutDataTypeStr=Inherit: Same as second input
  Subtract : Sum  Inputs=+-
  Out1 : Outport
  wires:
  Min/1 -> Out1/1
  Subtract/1 -> PID Controller/1
  Add2/1 -> Min/2
  Gain2/1 -> Add2/1
  I_Ref/1 -> Subtract/1
  Delta_Max/1 -> Min/1
  Delta_Est/1 -> Add2/2
  PID Controller/1 -> Gain2/1
  I_Load/1 -> Subtract/2

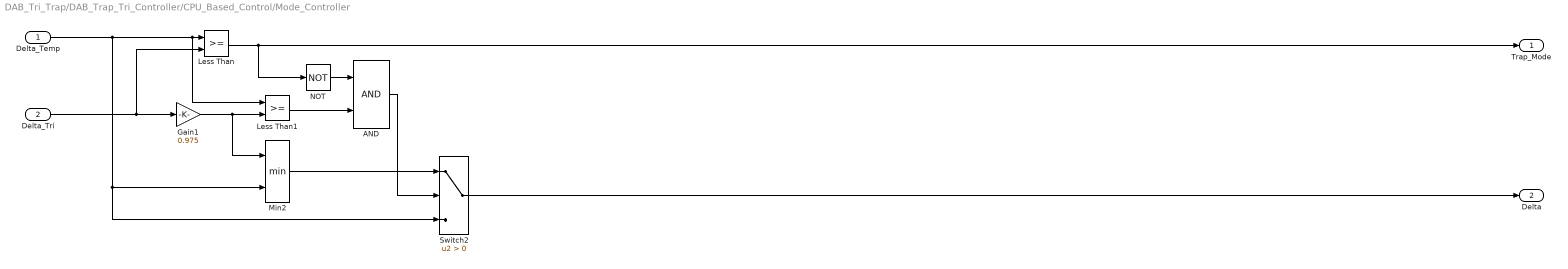
== system DAB_Tri_Trap/DAB_Trap_Tri_Controller/CPU_Based_Control/Mode_Controller ==
  Delta_Temp : Inport
  Delta_Tri : Inport  Port=2
  AND : Logic  IconShape=distinctive  AllPortsSameDT=off  OutDataTypeStr=boolean
  Gain1 : Gain  Gain=0.975
  Less Than : RelationalOperator  OutDataTypeStr=boolean  RndMeth=Simplest  InputSameDT=off
  Less Than1 : RelationalOperator  OutDataTypeStr=boolean  RndMeth=Simplest  InputSameDT=off
  Min2 : MinMax  Inputs=2
  NOT : Logic  Operator=NOT  IconShape=distinctive  AllPortsSameDT=off  OutDataTypeStr=boolean
  Switch2 : Switch  Criteria=u2 > Threshold  SaturateOnIntegerOverflow=off  InputSameDT=off
  Trap_Mode : Outport
  Delta : Outport  Port=2
  wires:
  Less Than/1 -> Trap_Mode/1, NOT/1
  Min2/1 -> Switch2/1
  Delta_Tri/1 -> Gain1/1, Less Than/2
  Gain1/1 -> Min2/1, Less Than1/2
  Delta_Temp/1 -> Less Than1/1, Less Than/1, Switch2/3, Min2/2
  Switch2/1 -> Delta/1
  NOT/1 -> AND/1
  AND/1 -> Switch2/2
  Less Than1/1 -> AND/2

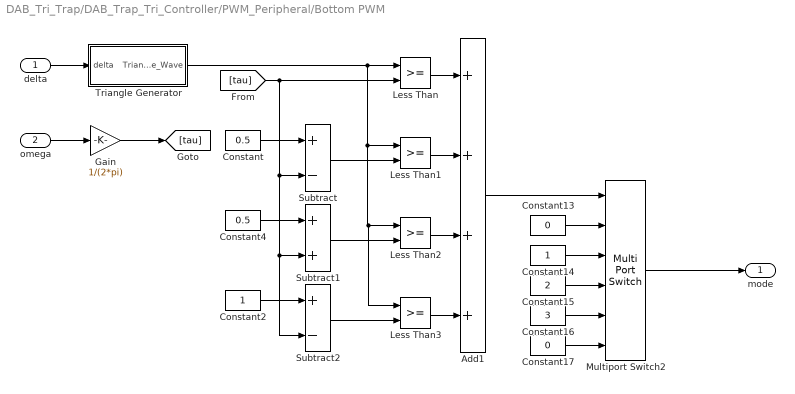
== system DAB_Tri_Trap/DAB_Trap_Tri_Controller/PWM_Peripheral/Bottom PWM ==
  delta : Inport
  omega : Inport  Port=2
  Add1 : Sum  Inputs=++++  AccumDataTypeStr=int8
  Constant : Constant  Value=0.5  SampleTime=ts_pwm
  Constant13 : Constant  Value=0  OutDataTypeStr=int16  SampleTime=ts_pwm
  Constant14 : Constant  OutDataTypeStr=int16  SampleTime=ts_pwm
  Constant15 : Constant  Value=2  OutDataTypeStr=int16  SampleTime=ts_pwm
  Constant16 : Constant  Value=3  OutDataTypeStr=int16  SampleTime=ts_pwm
  Constant17 : Constant  Value=0  OutDataTypeStr=int16  SampleTime=ts_pwm
  Constant2 : Constant  SampleTime=ts_pwm
  Constant4 : Constant  Value=0.5  SampleTime=ts_pwm
  Gain : Gain  Gain=1/(2*pi)
  Less Than{,1..3} (4 alike) : RelationalOperator  OutDataTypeStr=boolean  RndMeth=Simplest  InputSameDT=off
  Multiport Switch2 : MultiPortSwitch  DataPortOrder=Zero-based contiguous  Inputs=5  zeroidx=on  SaturateOnIntegerOverflow=off  InputSameDT=off
  Subtract : Sum  Inputs=+-
  Subtract1 : Sum
  Subtract2 : Sum  Inputs=+-
  Triangle Generator : Subsystem
  mode : Outport
  wires:
  Constant17/1 -> Multiport Switch2/6
  Constant16/1 -> Multiport Switch2/5
  Constant15/1 -> Multiport Switch2/4
  Constant14/1 -> Multiport Switch2/3
  Constant13/1 -> Multiport Switch2/2
  Gain/1 -> [tau]
  Less Than1/1 -> Add1/2
  Less Than3/1 -> Add1/4
  Add1/1 -> Multiport Switch2/1
  Subtract/1 -> Less Than1/2
  Constant4/1 -> Subtract1/1
  Constant/1 -> Subtract/1
  [tau] -> Less Than/2, Subtract/2, Subtract1/2, Subtract2/2
  Subtract2/1 -> Less Than3/2
  Less Than2/1 -> Add1/3
  Constant2/1 -> Subtract2/1
  Subtract1/1 -> Less Than2/2
  Less Than/1 -> Add1/1
  omega/1 -> Gain/1
  delta/1 -> Triangle Generator/1(delta)
  Triangle Generator/1(Triangle_Wave) -> Less Than/1, Less Than1/1, Less Than2/1, Less Than3/1
  Multiport Switch2/1 -> mode/1

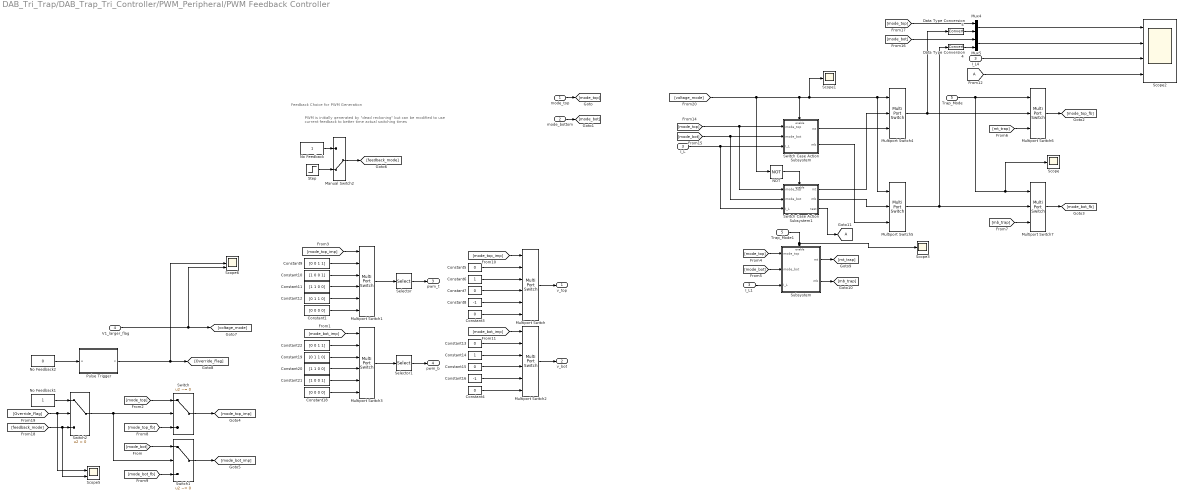
== system DAB_Tri_Trap/DAB_Trap_Tri_Controller/PWM_Peripheral/PWM Feedback Controller ==
  note: PWM is initially generated by "dead reckoning" but can be modified to use current feedback to better time actual switching times
  note: Feedback Choice for PWM Generation
  mode_top : Inport
  mode_bottom : Inport  Port=2
  I_L : Inport  Port=3
  V1_larger_flag : Inport  Port=4
  Trap_Mode : Inport  Port=5
  Constant1 : Constant  Value=[0 0 0 0]  SampleTime=ts_pwm
  Constant10 : Constant  Value=[1 0 0 1]  SampleTime=ts_pwm
  Constant11 : Constant  Value=[1 1 0 0]  SampleTime=ts_pwm
  Constant12 : Constant  Value=[0 1 1 0]  SampleTime=ts_pwm
  Constant{3..5,7,13,15} (6 alike) : Constant  Value=0  OutDataTypeStr=int16  SampleTime=ts_pwm
  Constant14 : Constant  OutDataTypeStr=int16  SampleTime=ts_pwm
  Constant16 : Constant  Value=-1  OutDataTypeStr=int16  SampleTime=ts_pwm
  Constant18 : Constant  Value=[0 0 0 0]  SampleTime=ts_pwm
  Constant19 : Constant  Value=[0 1 1 0]  SampleTime=ts_pwm
  Constant20 : Constant  Value=[1 1 0 0]  SampleTime=ts_pwm
  Constant21 : Constant  Value=[1 0 0 1]  SampleTime=ts_pwm
  Constant22 : Constant  Value=[0 0 1 1]  SampleTime=ts_pwm
  Constant6 : Constant  OutDataTypeStr=int16  SampleTime=ts_pwm
  Constant8 : Constant  Value=-1  OutDataTypeStr=int16  SampleTime=ts_pwm
  Constant9 : Constant  Value=[0 0 1 1]  SampleTime=ts_pwm
  Data Type Conversion4 : DataTypeConversion  SaturateOnIntegerOverflow=off  RndMeth=Floor
  Data Type Conversion5 : DataTypeConversion  SaturateOnIntegerOverflow=off  RndMeth=Floor
  From12 : From  TagVisibility=global
  Goto11 : Goto  TagVisibility=global
  I_L1 : InportShadow  Port=3
  I_L4 : InportShadow  Port=3
  Manual Switch2 : ManualSwitch  CurrentSetting=0
  Multiport Switch{,1..3} (4 alike) : MultiPortSwitch  DataPortOrder=Zero-based contiguous  Inputs=4  DataPortForDefault=Additional data port  zeroidx=on  SaturateOnIntegerOverflow=off  InputSameDT=off
  Multiport Switch{4..7} (4 alike) : MultiPortSwitch  DataPortOrder=Zero-based contiguous  Inputs=2  zeroidx=on  SaturateOnIntegerOverflow=off  InputSameDT=off
  Mux4 : Mux  Inputs=2
  Mux5 : Mux  Inputs=2
  NOT : Logic  Operator=NOT  IconShape=distinctive  AllPortsSameDT=off  OutDataTypeStr=boolean
  No Feedback : Constant
  No Feedback1 : Constant
  No Feedback2 : Constant  Value=0
  Pulse Trigger : Subsystem
  Scope : Scope
  Scope1 : Scope
  Scope2 : Scope  NumInputPorts=4
  Scope3 : Scope
  Scope5 : Scope  NumInputPorts=2
  Scope6 : Scope  NumInputPorts=3
  Selector : Selector  InputPortWidth=4  IndexOptions=Index vector (dialog)  Indices=[1 3 2 4]  OutputSizes=1
  Selector1 : Selector  InputPortWidth=4  IndexOptions=Index vector (dialog)  Indices=[2 4 1 3]  OutputSizes=1
  Step : Step  Time=1/fsw  Before=1  After=0  SampleTime=0
  Subsystem : Subsystem
  Switch : Switch  Criteria=u2 ~= 0  SaturateOnIntegerOverflow=off  InputSameDT=off
  Switch Case Action Subsystem : Subsystem  TreatAsAtomicUnit=on
  Switch Case Action Subsystem1 : Subsystem  TreatAsAtomicUnit=on
  Switch1 : Switch  Criteria=u2 ~= 0  SaturateOnIntegerOverflow=off  InputSameDT=off
  Switch2 : Switch  Criteria=u2 > Threshold  SaturateOnIntegerOverflow=off  InputSameDT=off
  Trap_Mode1 : InportShadow  Port=5
  v_top : Outport
  v_bot : Outport  Port=2
  pwm_t : Outport  Port=3
  pwm_b : Outport  Port=4
  wires:
  Constant16/1 -> Multiport Switch2/5
  Constant7/1 -> Multiport Switch/4
  Constant13/1 -> Multiport Switch2/2
  Multiport Switch1/1 -> Selector/1
  mode_bottom/1 -> [mode_bot]
  [mode_top_imp] -> Multiport Switch/1
  mode_top/1 -> [mode_top]
  Selector1/1 -> pwm_b/1
  Constant6/1 -> Multiport Switch/3
  Constant15/1 -> Multiport Switch2/4
  Constant14/1 -> Multiport Switch2/3
  Constant11/1 -> Multiport Switch1/4
  [mode_bot_imp] -> Multiport Switch3/1
  Constant18/1 -> Multiport Switch3/6
  [mode_top_imp] -> Multiport Switch1/1
  Constant5/1 -> Multiport Switch/2
  Constant3/1 -> Multiport Switch/6
  Constant8/1 -> Multiport Switch/5
  Constant1/1 -> Multiport Switch1/6
  Constant9/1 -> Multiport Switch1/2
  Selector/1 -> pwm_t/1
  [mode_bot_imp] -> Multiport Switch2/1
  Constant10/1 -> Multiport Switch1/3
  Constant12/1 -> Multiport Switch1/5
  Constant22/1 -> Multiport Switch3/2
  Multiport Switch3/1 -> Selector1/1
  Constant20/1 -> Multiport Switch3/4
  Constant21/1 -> Multiport Switch3/5
  Constant19/1 -> Multiport Switch3/3
  Constant4/1 -> Multiport Switch2/6
  Multiport Switch2/1 -> v_bot/1
  Multiport Switch/1 -> v_top/1
  [mode_top] -> Switch/1
  No Feedback/1 -> Manual Switch2/1
  Manual Switch2/1 -> [feedback_mode]
  [mode_bot] -> Switch1/1
  [mode_top_fb] -> Switch/3
  [mode_bot_fb] -> Switch1/3
  Switch/1 -> [mode_top_imp]
  Switch1/1 -> [mode_bot_imp]
  Step/1 -> Manual Switch2/2
  [voltage_mode] -> NOT/1, Switch Case Action Subsystem/Enable, Scope1/1, Multiport Switch5/1, Multiport Switch4/1
  [mode_bot] -> Switch Case Action Subsystem1/2(mode_bot), Switch Case Action Subsystem/2(mode_bot)
  [mode_top] -> Switch Case Action Subsystem1/1(mode_top), Switch Case Action Subsystem/1(mode_top)
  I_L/1 -> Switch Case Action Subsystem1/3(I_L), Switch Case Action Subsystem/3(I_L)
  [mode_bot] -> Mux5/1
  [mode_top] -> Mux4/1
  Mux4/1 -> Scope2/1
  Data Type Conversion4/1 -> Mux5/2
  Mux5/1 -> Scope2/2
  Data Type Conversion5/1 -> Mux4/2
  Multiport Switch4/1 -> Multiport Switch6/2, Data Type Conversion5/1
  Multiport Switch5/1 -> Multiport Switch7/2, Data Type Conversion4/1
  Switch Case Action Subsystem/1(mt) -> Multiport Switch4/3
  Switch Case Action Subsystem/2(mb) -> Multiport Switch5/3
  Switch Case Action Subsystem1/1(mt) -> Multiport Switch4/2
  Switch Case Action Subsystem1/2(mb) -> Multiport Switch5/2
  NOT/1 -> Switch Case Action Subsystem1/Enable
  I_L4/1 -> Scope2/3
  Switch2/1 -> Switch1/2, Switch/2
  [feedback_mode] -> Scope5/2, Switch2/3
  V1_larger_flag/1 -> [voltage_mode], Scope6/3
  No Feedback1/1 -> Switch2/1
  Pulse Trigger/1(x) -> Scope6/2, [Override_Flag]
  [Override_Flag] -> Scope5/1, Switch2/2
  [mode_top] -> Subsystem/1(mode_top)
  [mode_bot] -> Subsystem/2(mode_bot)
  I_L1/1 -> Subsystem/3(I_L)
  Multiport Switch6/1 -> [mode_top_fb]
  Multiport Switch7/1 -> [mode_bot_fb]
  Trap_Mode/1 -> Multiport Switch6/1, Scope/1, Multiport Switch7/1
  Trap_Mode1/1 -> Scope3/1, Subsystem/Enable
  Subsystem/1(mt) -> [mt_trap]
  Subsystem/2(mb) -> [mb_trap]
  [mt_trap] -> Multiport Switch6/3
  [mb_trap] -> Multiport Switch7/3
  From12/1 -> Scope2/4
  Switch Case Action Subsystem1/3(test) -> Goto11/1
  No Feedback2/1 -> Pulse Trigger/1(u)

== system DAB_Tri_Trap/DAB_Trap_Tri_Controller/PWM_Peripheral/Startup Enable ==
  Vnom1 : Inport
  Vnom2 : Inport  Port=2
  AND : Logic  IconShape=distinctive  AllPortsSameDT=off  OutDataTypeStr=boolean
  Compare To Zero : simulink/Logic and Bit Operations/Compare To Zero  relop===  OutDataTypeStr=boolean
  Compare To Zero1 : simulink/Logic and Bit Operations/Compare To Zero  relop===  OutDataTypeStr=boolean
  Constant1 : Constant  Value=true  SampleTime=ts_pwm
  Enabled Subsystem : Subsystem  TreatAsAtomicUnit=on
  Scope : Scope  NumInputPorts=3
  Out1 : Outport
  wires:
  AND/1 -> Enabled Subsystem/Enable
  Compare To Zero1/1 -> AND/2
  Enabled Subsystem/1(Out1) -> Scope/3, Out1/1
  Compare To Zero/1 -> AND/1
  Vnom2/1 -> Scope/2, Compare To Zero1/1
  Constant1/1 -> Enabled Subsystem/1(In1)
  Vnom1/1 -> Compare To Zero/1, Scope/1

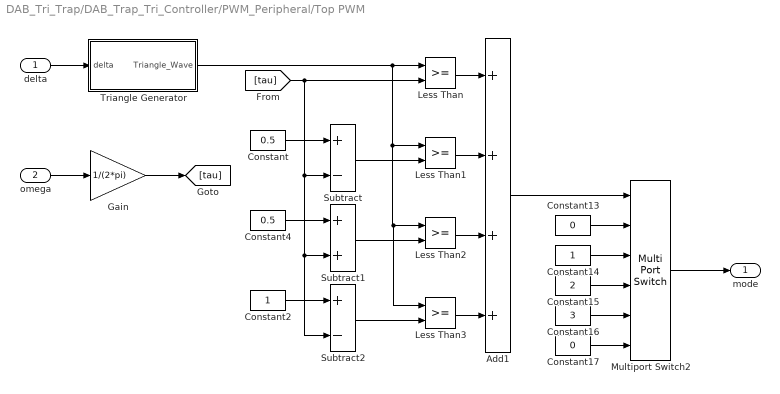
== system DAB_Tri_Trap/DAB_Trap_Tri_Controller/PWM_Peripheral/Top PWM ==
  delta : Inport
  omega : Inport  Port=2
  Add1 : Sum  Inputs=++++  AccumDataTypeStr=int8
  Constant : Constant  Value=0.5  SampleTime=ts_pwm
  Constant13 : Constant  Value=0  OutDataTypeStr=int16  SampleTime=ts_pwm
  Constant14 : Constant  OutDataTypeStr=int16  SampleTime=ts_pwm
  Constant15 : Constant  Value=2  OutDataTypeStr=int16  SampleTime=ts_pwm
  Constant16 : Constant  Value=3  OutDataTypeStr=int16  SampleTime=ts_pwm
  Constant17 : Constant  Value=0  OutDataTypeStr=int16  SampleTime=ts_pwm
  Constant2 : Constant  SampleTime=ts_pwm
  Constant4 : Constant  Value=0.5  SampleTime=ts_pwm
  Gain : Gain  Gain=1/(2*pi)
  Less Than{,1..3} (4 alike) : RelationalOperator  OutDataTypeStr=boolean  RndMeth=Simplest  InputSameDT=off
  Multiport Switch2 : MultiPortSwitch  DataPortOrder=Zero-based contiguous  Inputs=5  zeroidx=on  SaturateOnIntegerOverflow=off  InputSameDT=off
  Subtract : Sum  Inputs=+-
  Subtract1 : Sum
  Subtract2 : Sum  Inputs=+-
  Triangle Generator : Subsystem
  mode : Outport
  wires:
  Multiport Switch2/1 -> mode/1
  Triangle Generator/1(Triangle_Wave) -> Less Than3/1, Less Than2/1, Less Than1/1, Less Than/1
  delta/1 -> Triangle Generator/1(delta)
  omega/1 -> Gain/1
  Less Than/1 -> Add1/1
  Subtract1/1 -> Less Than2/2
  Constant2/1 -> Subtract2/1
  Less Than2/1 -> Add1/3
  Subtract2/1 -> Less Than3/2
  [tau] -> Subtract2/2, Subtract1/2, Subtract/2, Less Than/2
  Constant/1 -> Subtract/1
  Constant4/1 -> Subtract1/1
  Subtract/1 -> Less Than1/2
  Add1/1 -> Multiport Switch2/1
  Less Than3/1 -> Add1/4
  Less Than1/1 -> Add1/2
  Gain/1 -> [tau]
  Constant13/1 -> Multiport Switch2/2
  Constant14/1 -> Multiport Switch2/3
  Constant15/1 -> Multiport Switch2/4
  Constant16/1 -> Multiport Switch2/5
  Constant17/1 -> Multiport Switch2/6

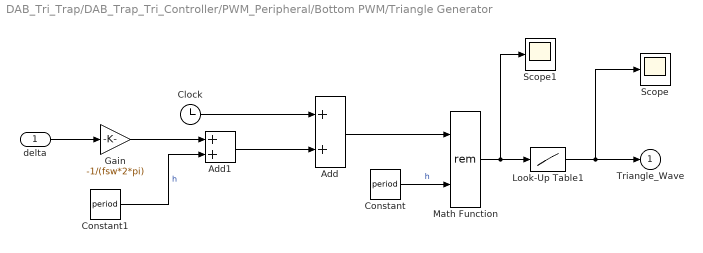
== system DAB_Tri_Trap/DAB_Trap_Tri_Controller/PWM_Peripheral/Bottom PWM/Triangle Generator ==
  delta : Inport
  Add : Sum
  Add1 : Sum
  Clock : Clock
      settings: DisableCoverage=on
  Constant : Constant  Value=period  SampleTime=ts_pwm
  Constant1 : Constant  Value=period  SampleTime=ts_pwm
  Gain : Gain  Gain=-1/(fsw*2*pi)
  Look-Up Table1 : Lookup_n-D  DisableCoverage=on  NumberOfTableDimensions=1  BreakpointsForDimension1=[0 1]*period  BreakpointsForDimension3=[5, 7]  Table=[0 1]  InternalRulePriority=Speed  SaturateOnIntegerOverflow=on
  Math Function : Math  DisableCoverage=on  Operator=rem
  Scope : Scope
  Scope1 : Scope
  Triangle_Wave : Outport
  wires:
  Constant1/1 -> Add1/2  "h"
  Add1/1 -> Add/2
  Gain/1 -> Add1/1
  Constant/1 -> Math Function/2  "h"
  Math Function/1 -> Look-Up Table1/1, Scope1/1
  delta/1 -> Gain/1
  Add/1 -> Math Function/1
  Look-Up Table1/1 -> Triangle_Wave/1, Scope/1
  Clock/1 -> Add/1

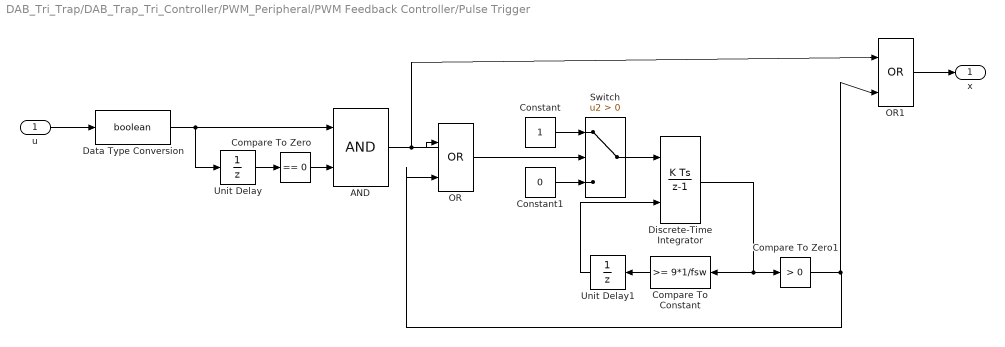
== system DAB_Tri_Trap/DAB_Trap_Tri_Controller/PWM_Peripheral/PWM Feedback Controller/Pulse Trigger ==
  u : Inport
  AND : Logic  IconShape=distinctive  AllPortsSameDT=off  OutDataTypeStr=boolean
  Compare To Constant : simulink/Logic and Bit Operations/Compare To Constant  relop=>=  const=9*1/fsw  OutDataTypeStr=boolean
  Compare To Zero : simulink/Logic and Bit Operations/Compare To Zero  relop===  OutDataTypeStr=boolean
  Compare To Zero1 : simulink/Logic and Bit Operations/Compare To Zero  relop=>  OutDataTypeStr=boolean
  Constant : Constant  SampleTime=-1
  Constant1 : Constant  Value=0  SampleTime=-1
  Data Type Conversion : DataTypeConversion  OutDataTypeStr=boolean  SaturateOnIntegerOverflow=off  RndMeth=Floor
  Discrete-Time Integrator : DiscreteIntegrator  ExternalReset=rising  SampleTime=-1  ICPrevOutput=DiscIntNeverNeededParam  ICPrevScaledInput=DiscIntNeverNeededParam
  OR : Logic  Operator=OR  IconShape=distinctive  AllPortsSameDT=off  OutDataTypeStr=boolean
  OR1 : Logic  Operator=OR  IconShape=distinctive  AllPortsSameDT=off  OutDataTypeStr=boolean
  Switch : Switch  Criteria=u2 > Threshold  SaturateOnIntegerOverflow=off  InputSameDT=off
  Unit Delay : UnitDelay  SampleTime=-1  HasFrameUpgradeWarning=on
  Unit Delay1 : UnitDelay  SampleTime=-1  HasFrameUpgradeWarning=on
  x : Outport
  wires:
  Unit Delay/1 -> Compare To Zero/1
  Compare To Zero/1 -> AND/2
  Compare To Constant/1 -> Unit Delay1/1
  Constant/1 -> Switch/1
  Discrete-Time Integrator/1 -> Compare To Constant/1, Compare To Zero1/1
  Constant1/1 -> Switch/3
  Compare To Zero1/1 -> OR1/2, OR/2
  Data Type Conversion/1 -> Unit Delay/1, AND/1
  OR/1 -> Switch/2
  AND/1 -> OR1/1, OR/1
  Switch/1 -> Discrete-Time Integrator/1
  u/1 -> Data Type Conversion/1
  Unit Delay1/1 -> Discrete-Time Integrator/2
  OR1/1 -> x/1

== system DAB_Tri_Trap/DAB_Trap_Tri_Controller/PWM_Peripheral/PWM Feedback Controller/Subsystem ==
  mode_top : Inport
  mode_bot : Inport  Port=2
  I_L : Inport  Port=3
  Enable : EnablePort
  Commutation Logic : Stateflow chart  TreatAsAtomicUnit=on
      settings: PortSchema="{\"entries\":[{\"content\":{\"sides\":[{\"content\":{\"connectorIds\":[\"In1\",\"In2\",\"In3\"]},\"type\":\"ConnectorPlacement.EquallySpacedRectSide\",\"uuid\":\"5493268e-b5c1-481e-98b7-42f968410dd3\"},{\"content\":{\"connectorIds\":[\"Out2\",\"Out3\",\"Out1\"],\"side\":\"RIGHT\"},\"type\":\"ConnectorPlacement.EquallySpacedRectSide\",\"uuid\":\"7b9bf0a8-4a9d-43f2-9fb6-d72373a79e7b\"},{\"content\":{\"connectorIds\":[],\"side\":\"TOP\"},\"type\":\"ConnectorPlacement.EquallySpacedRectSide\",\"uuid\":\"41bee1fe-d97f-41a9-b619-764ff8ca4954\"}]},\"type\":\"ConnectorPlacement.EquallySpacedConnector\",\"uuid\":\"6120a2cf-ea2a-45c2-bb23-5f4b1caef0a1\"}],\"packageUris\":[\"http://schema.mathworks.com/mf0/Connector/R2020b\"],\"version\":\"1.0\"}"
  Terminator : Terminator
  mt : Outport
  mb : Outport  Port=2
  wires:
  Commutation Logic/1(test) -> Terminator/1
  mode_top/1 -> Commutation Logic/1(mode_top)
  Commutation Logic/3(mb) -> mb/1
  I_L/1 -> Commutation Logic/3(I_L)
  mode_bot/1 -> Commutation Logic/2(mode_bot)
  Commutation Logic/2(mt) -> mt/1

== system DAB_Tri_Trap/DAB_Trap_Tri_Controller/PWM_Peripheral/PWM Feedback Controller/Switch Case Action Subsystem ==
  mode_top : Inport
  mode_bot : Inport  Port=2
  I_L : Inport  Port=3
  Enable : EnablePort
  Commutation Logic for V1 > V1 : Stateflow chart  TreatAsAtomicUnit=on
  Scope : Scope
  Terminator2 : Terminator
  mt : Outport
  mb : Outport  Port=2
  wires:
  Commutation Logic for V1 > V1/1(test) -> Terminator2/1
  mode_top/1 -> Commutation Logic for V1 > V1/1(mode_top)
  Commutation Logic for V1 > V1/2(mt) -> Scope/1, mt/1
  Commutation Logic for V1 > V1/3(mb) -> mb/1
  mode_bot/1 -> Commutation Logic for V1 > V1/2(mode_bot)
  I_L/1 -> Commutation Logic for V1 > V1/3(I_L)

== system DAB_Tri_Trap/DAB_Trap_Tri_Controller/PWM_Peripheral/PWM Feedback Controller/Switch Case Action Subsystem1 ==
  mode_top : Inport
  mode_bot : Inport  Port=2
  I_L : Inport  Port=3
  Enable : EnablePort
  Commutation Logic : Stateflow chart  TreatAsAtomicUnit=on
      settings: PortSchema="{\"entries\":[{\"content\":{\"sides\":[{\"content\":{\"connectorIds\":[\"In1\",\"In2\",\"In3\"]},\"type\":\"ConnectorPlacement.EquallySpacedRectSide\",\"uuid\":\"5493268e-b5c1-481e-98b7-42f968410dd3\"},{\"content\":{\"connectorIds\":[\"Out2\",\"Out3\",\"Out1\"],\"side\":\"RIGHT\"},\"type\":\"ConnectorPlacement.EquallySpacedRectSide\",\"uuid\":\"7b9bf0a8-4a9d-43f2-9fb6-d72373a79e7b\"},{\"content\":{\"connectorIds\":[],\"side\":\"TOP\"},\"type\":\"ConnectorPlacement.EquallySpacedRectSide\",\"uuid\":\"41bee1fe-d97f-41a9-b619-764ff8ca4954\"}]},\"type\":\"ConnectorPlacement.EquallySpacedConnector\",\"uuid\":\"6120a2cf-ea2a-45c2-bb23-5f4b1caef0a1\"}],\"packageUris\":[\"http://schema.mathworks.com/mf0/Connector/R2020b\"],\"version\":\"1.0\"}"
  mt : Outport
  mb : Outport  Port=2
  test : Outport  Port=3
  wires:
  I_L/1 -> Commutation Logic/3(I_L)
  Commutation Logic/1(test) -> test/1
  Commutation Logic/2(mt) -> mt/1
  Commutation Logic/3(mb) -> mb/1
  mode_bot/1 -> Commutation Logic/2(mode_bot)
  mode_top/1 -> Commutation Logic/1(mode_top)

== system DAB_Tri_Trap/DAB_Trap_Tri_Controller/PWM_Peripheral/Startup Enable/Enabled Subsystem ==
  In1 : Inport
  Enable : EnablePort
  Out1 : Outport  OutDataTypeStr=boolean  InitialOutput=[false]
  wires:
  In1/1 -> Out1/1

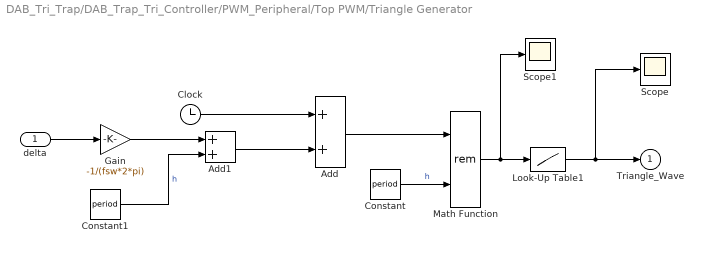
== system DAB_Tri_Trap/DAB_Trap_Tri_Controller/PWM_Peripheral/Top PWM/Triangle Generator ==
  delta : Inport
  Add : Sum
  Add1 : Sum
  Clock : Clock
      settings: DisableCoverage=on
  Constant : Constant  Value=period  SampleTime=ts_pwm
  Constant1 : Constant  Value=period  SampleTime=ts_pwm
  Gain : Gain  Gain=-1/(fsw*2*pi)
  Look-Up Table1 : Lookup_n-D  DisableCoverage=on  NumberOfTableDimensions=1  BreakpointsForDimension1=[0 1]*period  BreakpointsForDimension3=[5, 7]  Table=[0 1]  InternalRulePriority=Speed  SaturateOnIntegerOverflow=on
  Math Function : Math  DisableCoverage=on  Operator=rem
  Scope : Scope
  Scope1 : Scope
  Triangle_Wave : Outport
  wires:
  Clock/1 -> Add/1
  Look-Up Table1/1 -> Scope/1, Triangle_Wave/1
  Add/1 -> Math Function/1
  delta/1 -> Gain/1
  Math Function/1 -> Scope1/1, Look-Up Table1/1
  Constant/1 -> Math Function/2  "h"
  Gain/1 -> Add1/1
  Add1/1 -> Add/2
  Constant1/1 -> Add1/2  "h"

== stateflow chart DAB_Tri_Trap/DAB_Trap_Tri_Controller/PWM_Peripheral/PWM Feedback Controller/Switch Case Action Subsystem1/Commutation Logic ==
  state A
    entry:
    test = 0;
    during:
    mt = mode_top;
    mb = mode_bot;
  state C
    entry:
    test = 2;
    mt = 1;
    mb = 1;
  state F
    entry:
    test = 5;
    mt = 3;
    mb = 3;
  state D
    entry:
    test = 3;
    during:
    mt = mode_top;
    mb = mode_bot;
  (default) -> A
  A -> C : [mode_top == 1 && mode_bot ==1]
  F -> A : [I_L >= 0]
  C -> D : [I_L <= 0]
  D -> F : [mode_top == 3 && mode_bot == 3]
  data: mode_top input; mode_bot input; test output int8; I_L input; mt output int16; mb output int16

== matlab function DAB_Tri_Trap/DAB_Trap_Tri_Controller/CPU_Based_Control/Delta_Max ==
  data: tau input; delta_Pmax output; fsw input; V1 input; V2 input; ex1 input; ex2 input; delta_Ptri output
function [delta_Pmax, delta_Ptri] = fcn(tau,fsw,V1,V2, ex1, ex2)

delta_Pmax = pi*(1-2*tau*fsw)/2*(ex1/ex2);

if V1 <= V2
    delta_Ptri = pi*(1-2*tau*fsw)/2*(1-V1/V2);
else
    delta_Ptri = pi*(1-2*tau*fsw)/2*(1-V2/V1);
end
